simulink model "Wheighted_mixer"  (R2016b)
settings: Solver=ode2  StartTime=0.0  StopTime=10.0  FixedStep=sample_time  RelTol=1e-3  EnableMultiTasking=on
InitFcn:
  | Parameters_physical_tiltrotor
  | Parameters_controllers_tiltrotor
undefined symbols (not defined in the file): Kinv, motor_ome_vs_throttle
settings Model: Creator=pela  LastModifiedBy=Mattia
settings DataIOCC: LimitDataPoints=on  SaveFormat=Array
settings OptimizationCC: LifeSpan=inf
settings DebuggingCC: SFUnexpectedBacktrackingDiag=warning  SFNoUnconditionalDefaultTransitionDiag=warning  SFExecutionAtInitializationDiag=none
settings HardwareCC: ProdBitPerPointer=32  ProdBitPerSizeT=32  ProdBitPerPtrDiffT=32  ProdLargestAtomicInteger=Long  ProdLargestAtomicFloat=Double  ProdIntDivRoundTo=Undefined  ProdWordSize=32  ProdHWDeviceType=ARM Compatible->ARM Cortex
settings ModelReferenceCC: PropagateSignalLabelsOutOfModel=off
settings RTWCC: GenCodeOnly=on  GenerateReport=on  BuildConfiguration=Faster Runs  LaunchReport=on  TargetLang=C++
settings GRTTargetCC: TargetLangStandard=C89/C90 (ANSI)  GeneratePreprocessorConditionals=Disable all  MatFileLogging=off  MultiInstanceERTCode=on  CodeInterfacePackaging=C++ class
settings ConfigComp: CovMetricSettings=dw  CovHtmlReporting=on  CovSaveCumulativeToWorkspaceVar=on  CovSaveSingleToWorkspaceVar=on  CovExternalEMLEnable=off

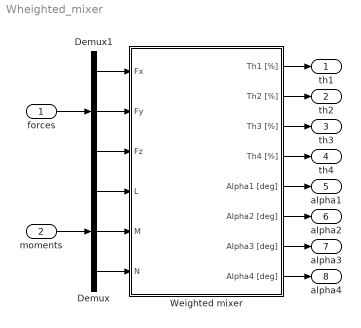
== system Wheighted_mixer ==
  forces : Inport
  moments : Inport  Port=2
  Demux : Demux  Outputs=3
  Demux1 : Demux  Outputs=3
  Weighted mixer : Subsystem
  th1 : Outport
  th2 : Outport  Port=2
  th3 : Outport  Port=3
  th4 : Outport  Port=4
  alpha1 : Outport  Port=5
  alpha2 : Outport  Port=6
  alpha3 : Outport  Port=7
  alpha4 : Outport  Port=8
  wires:
  Demux1/1 -> Weighted mixer/1(Fx)
  Demux/2 -> Weighted mixer/5(M)
  Demux/1 -> Weighted mixer/4(L)
  Demux/3 -> Weighted mixer/6(N)
  Weighted mixer/4(Th4 [%]) -> th4/1
  Weighted mixer/3(Th3 [%]) -> th3/1
  Weighted mixer/2(Th2 [%]) -> th2/1
  Weighted mixer/1(Th1 [%]) -> th1/1
  Weighted mixer/5(Alpha1 [deg]) -> alpha1/1
  Weighted mixer/6(Alpha2 [deg]) -> alpha2/1
  Weighted mixer/8(Alpha4 [deg]) -> alpha4/1
  Weighted mixer/7(Alpha3 [deg]) -> alpha3/1
  forces/1 -> Demux1/1
  Demux1/2 -> Weighted mixer/2(Fy)
  Demux1/3 -> Weighted mixer/3(Fz)
  moments/1 -> Demux/1

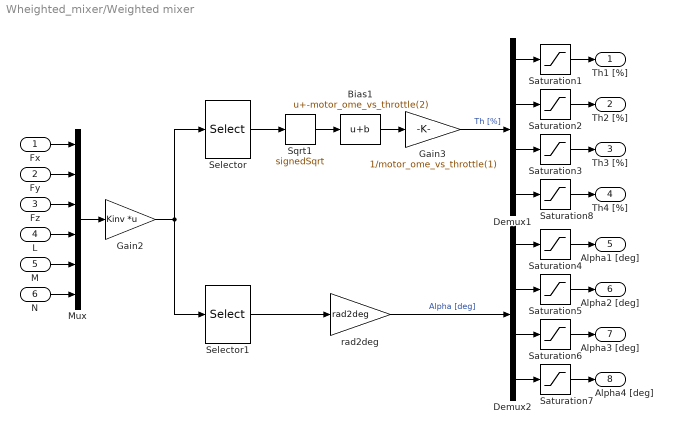
== system Wheighted_mixer/Weighted mixer ==
  Fx : Inport
  Fy : Inport  Port=2
  Fz : Inport  Port=3
  L : Inport  Port=4
  M : Inport  Port=5
  N : Inport  Port=6
  Bias1 : Bias  Bias=-motor_ome_vs_throttle(2)
  Demux1 : Demux
  Demux2 : Demux
  Gain2 : Gain  Gain=Kinv  Multiplication=Matrix(K*u)
  Gain3 : Gain  Gain=1/motor_ome_vs_throttle(1)
  Mux : Mux  Inputs=6
  Saturation{1..3,8} (4 alike) : Saturate  UpperLimit=100  LowerLimit=0
  Saturation{4..7} (4 alike) : Saturate  UpperLimit=45  LowerLimit=-45
  Selector : Selector  InputPortWidth=8  IndexOptions=Index vector (dialog)  Indices=[1 2 3 4]  OutputSizes=1
  Selector1 : Selector  InputPortWidth=8  IndexOptions=Index vector (dialog)  Indices=[5 6 7 8]  OutputSizes=1
  Sqrt1 : Sqrt  Operator=signedSqrt  SaturateOnIntegerOverflow=on
  rad2deg : Gain  Gain=rad2deg
  Th1 [%] : Outport
  Th2 [%] : Outport  Port=2
  Th3 [%] : Outport  Port=3
  Th4 [%] : Outport  Port=4
  Alpha1 [deg] : Outport  Port=5
  Alpha2 [deg] : Outport  Port=6
  Alpha3 [deg] : Outport  Port=7
  Alpha4 [deg] : Outport  Port=8
  wires:
  Saturation6/1 -> Alpha3 [deg]/1
  Demux2/1 -> Saturation4/1
  Demux2/3 -> Saturation6/1
  Sqrt1/1 -> Bias1/1
  Bias1/1 -> Gain3/1
  Demux2/2 -> Saturation5/1
  Demux2/4 -> Saturation7/1
  Saturation4/1 -> Alpha1 [deg]/1
  Saturation5/1 -> Alpha2 [deg]/1
  Saturation7/1 -> Alpha4 [deg]/1
  Fx/1 -> Mux/1
  Fy/1 -> Mux/2
  Fz/1 -> Mux/3
  L/1 -> Mux/4
  M/1 -> Mux/5
  N/1 -> Mux/6
  Selector/1 -> Sqrt1/1
  Selector1/1 -> rad2deg/1
  rad2deg/1 -> Demux2/1  "Alpha [deg]"
  Gain2/1 -> Selector1/1, Selector/1
  Mux/1 -> Gain2/1
  Demux1/3 -> Saturation3/1
  Demux1/2 -> Saturation2/1
  Demux1/4 -> Saturation8/1
  Demux1/1 -> Saturation1/1
  Saturation1/1 -> Th1 [%]/1
  Saturation2/1 -> Th2 [%]/1
  Saturation3/1 -> Th3 [%]/1
  Saturation8/1 -> Th4 [%]/1
  Gain3/1 -> Demux1/1  "Th [%]"
